simulink model "untitled3"  (R2025a)
settings: Solver=VariableStepAuto  StartTime=0.0  StopTime=1  RelTol=1e-3
libraries: spsMeanLib x5, spsCurrentMeasurementLib x2, spsDCVoltageSourceLib x2, spsSeriesRLCBranchLib x2, spsMultimeterLib x2, spsDCMachineLib x1, sps_lib x1, spsDiodeLib x1, spsGroundLib x1, spsMosfetLib x1, spsVoltageMeasurementLib x1
settings Model: Creator=user  LastModifiedBy=user

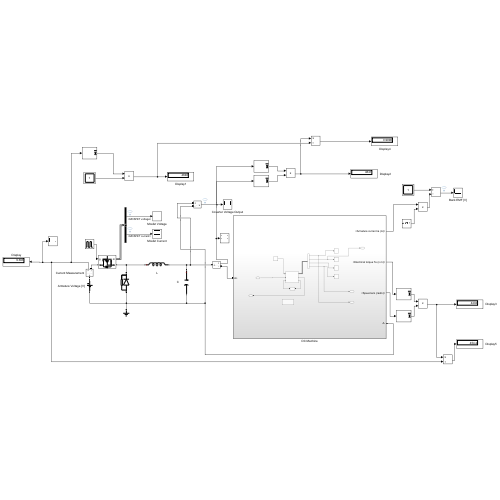
[thumbnail: Simulink's stored preview of the top-level diagram]
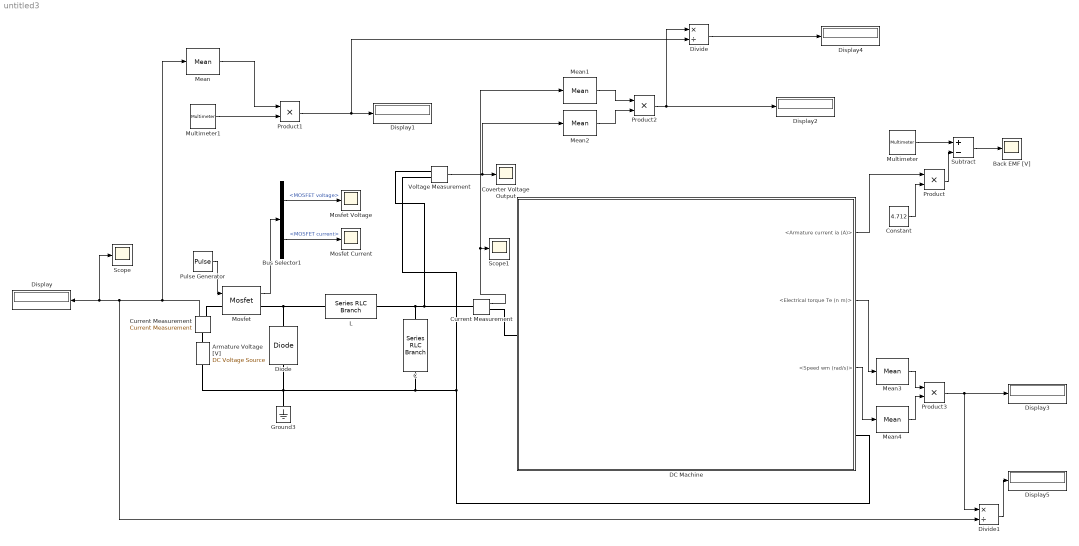
== system untitled3 ==
  " Current Measurement" : spsCurrentMeasurementLib/Current Measurement  PhasorSimulation=off  OutputType=Complex  PSBequivalent=0
   Display{,1..5} (6 alike) : Display
  Armature Voltage [V] : spsDCVoltageSourceLib/DC Voltage Source  Amplitude=500  Measurements=Voltage
  Back EMF [V] : Scope
      settings: DataLoggingVariableName=ScopeData4
  Bus Selector1 : BusSelector  OutputSignals=MOSFET voltage,MOSFET current
  C : spsSeriesRLCBranchLib/Series RLC Branch  LConnTagsString=__new0  RConnTagsString=__new0  BranchType=C  Resistance=50  Inductance=1e-3  SetiL0=off  InitialCurrent=0  Capacitance=1e-6  Setx0=off  InitialVoltage=0  Measurements=Branch voltage
  Constant : Constant  Value=4.712
  Coverter Voltage Output : Scope
      settings: ActiveDisplayYMinimum=-73.828497745517453  ActiveDisplayYMaximum=664.69206860870838  DataLoggingVariableName=ScopeData7
  Current Measurement : spsCurrentMeasurementLib/Current Measurement  PhasorSimulation=off  OutputType=Complex  PSBequivalent=0
  DC Machine : Subsystem
  Diode : spsDiodeLib/Diode  Ron=0.01  Lon=0  Vf=0.8  IC=0  UseSnubber=0  Rs=500  Cs=250e-9  Measurements=off
  Divide : Product  Inputs=*/
  Divide1 : Product  Inputs=*/
  Ground3 : spsGroundLib/Ground  LConnTagsString=a
  L : spsSeriesRLCBranchLib/Series RLC Branch  LConnTagsString=__new0  RConnTagsString=__new0  BranchType=L  Resistance=50  Inductance=0.1  SetiL0=off  InitialCurrent=0  Capacitance=1e-6  Setx0=off  InitialVoltage=0  Measurements=None
  Mean{,1..4} (5 alike) : spsMeanLib/Mean  Freq=60  Vinit=0  Ts=0
  Mosfet : spsMosfetLib/Mosfet  Ron=0.01  Lon=0  Rd=0.01  Vfd=1  IC=0  Rs=1e5  Cs=inf  Measurements=on
  Mosfet Current : Scope
      settings: DataLoggingVariableName=ScopeData6
  Mosfet Voltage : Scope
      settings: DataLoggingVariableName=ScopeData5
  Multimeter : spsMultimeterLib/Multimeter  L=2  sel=1  yselected={}  Gain=1  OutputType=Complex  PlotAtSimulationStop=off  PhasorSimulation=off
  Multimeter1 : spsMultimeterLib/Multimeter  L=2  sel=2  yselected={}  Gain=1  OutputType=Complex  PlotAtSimulationStop=off  PhasorSimulation=off
  Product{,1..3} (4 alike) : Product
  Pulse Generator : DiscretePulseGenerator  PulseType=Time based  Period=1\25000  PulseWidth=70
  Scope : Scope
      settings: DataLoggingVariableName=ScopeData8
  Scope1 : Scope
      settings: DataLoggingVariableName=ScopeData9
  Subtract : Sum  Inputs=+-
  Voltage Measurement : spsVoltageMeasurementLib/Voltage Measurement  PhasorSimulation=off  OutputType=Complex  PSBequivalent=0
  wires:
  Subtract/1 -> Back EMF [V]/1
  Multimeter/1 -> Subtract/1
  Product/1 -> Subtract/2
  Constant/1 -> Product/2
  Pulse Generator/1 -> Mosfet/1
  Mosfet/1 -> Bus Selector1/1
  Bus Selector1/2 -> Mosfet Current/1  "<MOSFET current>"
  Bus Selector1/1 -> Mosfet Voltage/1  "<MOSFET voltage>"
  Voltage Measurement/1 -> Coverter Voltage Output/1, Mean2/1
  Current Measurement/1 -> Mean1/1, Scope1/1
  Multimeter1/1 -> Product1/2
  Mean/1 -> Product1/1
  Product1/1 -> Divide/2, " Display1"/1
  Mean1/1 -> Product2/1
  Mean2/1 -> Product2/2
  Product2/1 -> Divide/1, " Display2"/1
  Mean3/1 -> Product3/1
  Mean4/1 -> Product3/2
  Divide/1 -> " Display4"/1
  Product3/1 -> Divide1/1, " Display3"/1
  " Current Measurement"/1 -> Divide1/2, Scope/1, " Display"/1, Mean/1
  Divide1/1 -> " Display5"/1
  DC Machine/1(<Armature current ia (A)>) -> Product/1
  DC Machine/2(<Electrical torque Te (n m)>) -> Mean3/1
  DC Machine/3(<Speed wm (rad/s)>) -> Mean4/1
  connections:
  L/RConn1 -- Current Measurement/LConn1 -- Voltage Measurement/LConn1 -- C/LConn1
  Mosfet/RConn1 -- Diode/RConn1 -- L/LConn1
  Armature Voltage [V]/LConn1 -- Diode/LConn1 -- Ground3/LConn1 -- DC Machine/RConn1 -- Voltage Measurement/LConn2 -- C/RConn1
  " Current Measurement"/RConn1 -- Mosfet/LConn1
  Armature Voltage [V]/RConn1 -- " Current Measurement"/LConn1
  DC Machine/LConn1 -- Current Measurement/RConn1

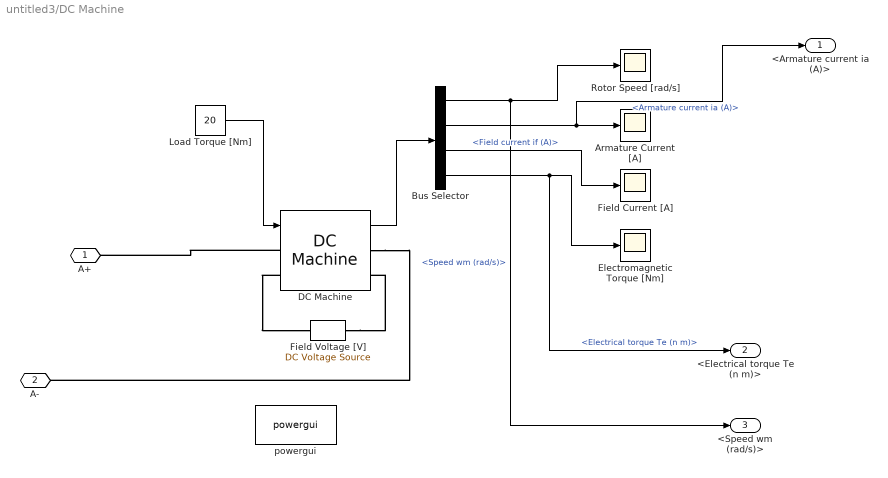
== system untitled3/DC Machine ==
  Armature Current [A] : Scope
      settings: ActiveDisplayYMinimum=-8.0571894742010279  ActiveDisplayYMaximum=72.558059932683747
  Bus Selector : BusSelector  OutputSignals=Speed wm (rad/s),Armature current ia (A),Field current if (A),Electrical torque Te (n m)
  DC Machine : spsDCMachineLib/DC Machine  PresetModel=05: 10HP 500V 1750RPM Field:300V  MechanicalLoad=Torque TL  FieldType=Wound  ShowDetailedParameters=on  MeasurementBus=off  RLa=[4.712 0.05277]  RLf=[180 71.47]  Laf=1.345  MachineConstant=Torque constant (N.m/A)  Ke=1.8  Kt=1.8  J=0.04251  Bm=0.003406  Tf=1.046  w0=1  Ifinit=1.66666666666667  TsPowergui=0  TsBlock=-1
  Electromagnetic Torque [Nm] : Scope
      settings: ActiveDisplayYMinimum=-18.06309201761119  ActiveDisplayYMaximum=162.65115756535241  DataLoggingVariableName=ScopeData3
  Field Current [A] : Scope
      settings: ActiveDisplayYMinimum=0.66666666666666674  ActiveDisplayYMaximum=2.666666666666667  DataLoggingVariableName=ScopeData2
  Field Voltage [V] : spsDCVoltageSourceLib/DC Voltage Source  Amplitude=300  Measurements=None
  Load Torque [Nm] : Constant  Value=20
  Rotor Speed [rad/s] : Scope
      settings: ActiveDisplayYMinimum=-27.888904195279913  ActiveDisplayYMaximum=253.54416094383731
  powergui : sps_lib/powergui  Priority=1  SimulationMode=Continuous  SampleTime=50e-6  frequency=60  Iterations=50  frequencyindice=0  Pbase=100e6  ErrMax=1e-4  UnitsV=kV  UnitsW=MW  buscounter=0  FunctionMessages=off  echomessages=off  EnableUseOfTLC=off  CurrentSourceSwitches=on  DisableSnubberDevices=off  DisableRonSwitches=off  DisableVfSwitches=off  DisplayEquations=off  AutomaticDiscreteSolvers=off  SolverType=Tustin/Backward Euler (TBE)  Interpol=off  ExternalGateDelay=off  methode=off  Ts=100  x0status=blocks  SPID=on  SwTol=0  HookPort=off  NonlinearTolerance=1e-4  nMaxIteration=100  ContinueOnMaxIteration=off  RestoreLinks=warning  ResistiveCurrentMeasurement=off  Frange=[0:2:500]  Ylog=off  Xlog=on  ShowGrid=off  save=off  variable=ZData  structure=0  ZoomFFT=off  StartTime=0.0  cycles=1  DisplayStyle=1  fundamental=60  FreqAxis=off  MaxFrequency=1000  frequencyindicesteady=1  RmsSteady=1  display=off
  A+ : PMIOPort  Side=Left
  A- : PMIOPort  Port=2  Side=Right
  <Armature current ia (A)> : Outport
  <Electrical torque Te (n m)> : Outport  Port=2
  <Speed wm (rad/s)> : Outport  Port=3
  wires:
  Bus Selector/4 -> <Electrical torque Te (n m)>/1, Electromagnetic Torque [Nm]/1  "<Electrical torque Te (n m)>"
  Load Torque [Nm]/1 -> DC Machine/1
  Bus Selector/2 -> <Armature current ia (A)>/1, Armature Current [A]/1  "<Armature current ia (A)>"
  Bus Selector/1 -> <Speed wm (rad/s)>/1, Rotor Speed [rad/s]/1  "<Speed wm (rad/s)>"
  Bus Selector/3 -> Field Current [A]/1  "<Field current if (A)>"
  DC Machine/1 -> Bus Selector/1
  connections:
  DC Machine/LConn2 -- Field Voltage [V]/RConn1
  Field Voltage [V]/LConn1 -- DC Machine/RConn2
  DC Machine/LConn1 -- A+/RConn1
  DC Machine/RConn1 -- A-/RConn1
